simulink model "week1_problem5"  (R2020b)
settings: Solver=VariableStepAuto  StartTime=0.0  StopTime=10.0  RelTol=1e-3
InitFcn:
  | R=20;
  | C=10*10^-6;
settings Model: Creator=gauri  LastModifiedBy=mluser

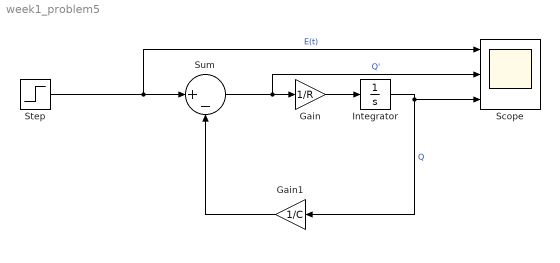
== system week1_problem5 ==
  Gain : Gain  Gain=1/R
  Gain1 : Gain  Gain=1/C
  Integrator : Integrator
  Scope : Scope  NumInputPorts=3
  Step : Step  SampleTime=0
  Sum : Sum  Inputs=|+-
  wires:
  Sum/1 -> Scope/2, Gain/1  "Q'"
  Gain/1 -> Integrator/1
  Integrator/1 -> Gain1/1, Scope/3  "Q"
  Gain1/1 -> Sum/2
  Step/1 -> Scope/1, Sum/1  "E(t)"
